simulink model "Integ_Model_Hepta_Runner"  (R2022a)
settings: configuration reference "VLS_Standard_Configuration" (kept outside this file)
libraries: simulink x1
settings Model: DataDictionary=Hepta_Integrated_SLDD.sldd  Creator=ahashem  LastModifiedBy=yli69
settings ConfigSetRef: SourceName=VLS_Standard_Configuration

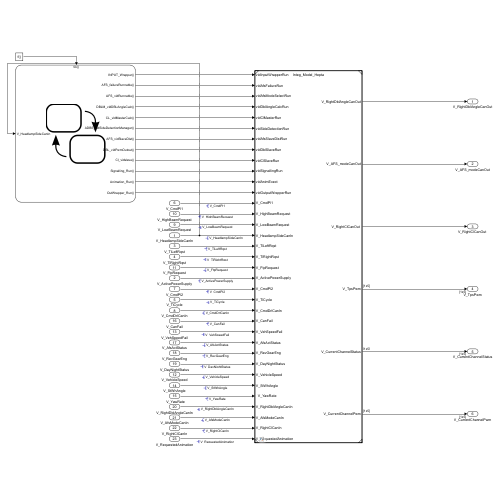
[thumbnail: Simulink's stored preview of the top-level diagram]
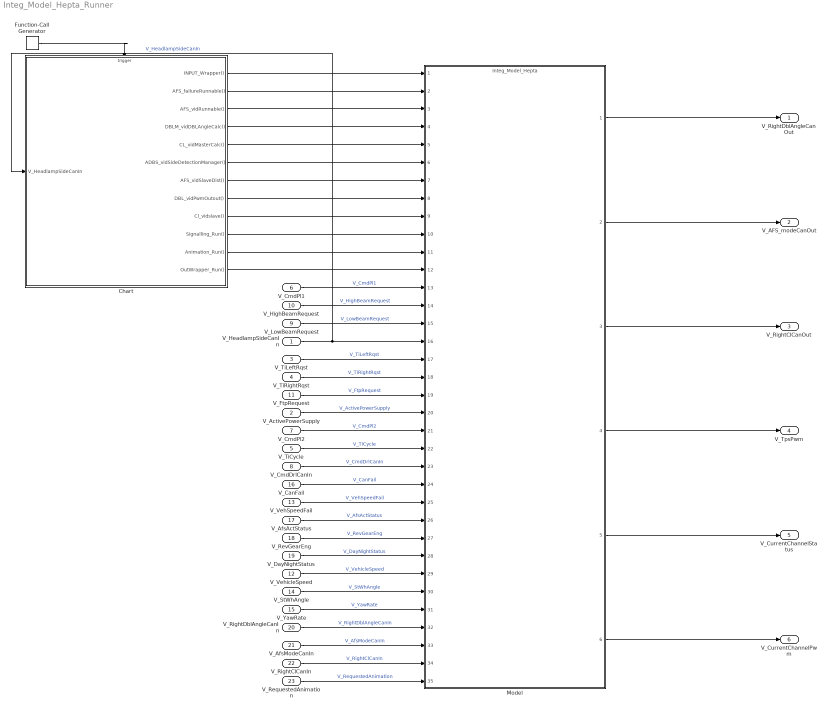
== system Integ_Model_Hepta_Runner ==
  V_HeadlampSideCanIn : Inport
  V_ActivePowerSupply : Inport  Port=2
  V_TiLeftRqst : Inport  Port=3
  V_TiRightRqst : Inport  Port=4
  V_TiCycle : Inport  Port=5
  V_CmdPl1 : Inport  Port=6
  V_CmdPl2 : Inport  Port=7
  V_CmdDrlCanIn : Inport  Port=8
  V_LowBeamRequest : Inport  Port=9
  V_HighBeamRequest : Inport  Port=10
  V_FtpRequest : Inport  Port=11
  V_VehicleSpeed : Inport  Port=12
  V_VehSpeedFail : Inport  Port=13
  V_StWhAngle : Inport  Port=14
  "  V_YawRate" : Inport  Port=15
  V_CanFail : Inport  Port=16
  V_AfsActStatus : Inport  Port=17
  V_RevGearEng : Inport  Port=18
  V_DayNightStatus : Inport  Port=19
  V_RightDblAngleCanIn : Inport  Port=20
  V_AfsModeCanIn : Inport  Port=21
  V_RightClCanIn : Inport  Port=22
  V_RequestedAnimation : Inport  Port=23
  Chart : Stateflow chart  TreatAsAtomicUnit=on
  Function-Call Generator : simulink/Ports & Subsystems/Function-Call Generator  sample_time=0.02  numberOfIterations=1  DisallowWideOutput=off
  Model : ModelReference  ModelNameDialog=Integ_Model_Hepta.slx  SimulationMode=Normal  ScheduleRates=on  ModelReferenceVersion=4.16
  V_RightDblAngleCanOut : Outport  VectorParamsAs1DForOutWhenUnconnected=off
  V_AFS_modeCanOut : Outport  Port=2  VectorParamsAs1DForOutWhenUnconnected=off
  "V_RightClCanOut " : Outport  Port=3  VectorParamsAs1DForOutWhenUnconnected=off
  V_TpsPwm : Outport  Port=4
  V_CurrentChannelStatus : Outport  Port=5
  V_CurrentChannelPwm : Outport  Port=6
  wires:
  Function-Call Generator/1 -> Chart/Trigger
  Chart/1(INPUT_Wrapper()) -> Model/1
  Chart/2(AFS_failureRunnable()) -> Model/2
  Chart/3(AFS_vidRunnable()) -> Model/3
  Chart/4(DBLM_vidDBLAngleCalc()) -> Model/4
  Chart/5(CL_vidMasterCalc()) -> Model/5
  Chart/6(ADBS_vidSideDetectionManager()) -> Model/6
  Chart/7(AFS_vidSlaveDist()) -> Model/7
  Chart/8(DBL_vidPwmOutout()) -> Model/8
  Chart/9(Cl_vidslave()) -> Model/9
  Chart/10(Signalling_Run()) -> Model/10
  Chart/11(Animation_Run()) -> Model/11
  V_HeadlampSideCanIn/1 -> Model/16, Chart/1(V_HeadlampSideCanIn)  "V_HeadlampSideCanIn"
  Model/1 -> V_RightDblAngleCanOut/1
  Model/2 -> V_AFS_modeCanOut/1
  Model/3 -> "V_RightClCanOut "/1
  Model/4 -> V_TpsPwm/1
  Model/5 -> V_CurrentChannelStatus/1
  Model/6 -> V_CurrentChannelPwm/1
  Chart/12(OutWrapper_Run()) -> Model/12
  V_CmdPl1/1 -> Model/13  "V_CmdPl1"
  V_HighBeamRequest/1 -> Model/14  "V_HighBeamRequest"
  V_LowBeamRequest/1 -> Model/15  "V_LowBeamRequest"
  V_TiLeftRqst/1 -> Model/17  "V_TiLeftRqst"
  V_TiRightRqst/1 -> Model/18  "V_TiRightRqst"
  V_FtpRequest/1 -> Model/19  "V_FtpRequest"
  V_ActivePowerSupply/1 -> Model/20  "V_ActivePowerSupply"
  V_CmdPl2/1 -> Model/21  "V_CmdPl2"
  V_TiCycle/1 -> Model/22  "V_TiCycle"
  V_CmdDrlCanIn/1 -> Model/23  "V_CmdDrlCanIn"
  V_CanFail/1 -> Model/24  "V_CanFail"
  V_VehSpeedFail/1 -> Model/25  "V_VehSpeedFail"
  V_AfsActStatus/1 -> Model/26  "V_AfsActStatus"
  V_RevGearEng/1 -> Model/27  "V_RevGearEng"
  V_DayNightStatus/1 -> Model/28  "V_DayNightStatus"
  V_VehicleSpeed/1 -> Model/29  "V_VehicleSpeed"
  V_StWhAngle/1 -> Model/30  "V_StWhAngle"
  "  V_YawRate"/1 -> Model/31  "V_YawRate"
  V_RightDblAngleCanIn/1 -> Model/32  "V_RightDblAngleCanIn"
  V_AfsModeCanIn/1 -> Model/33  "V_AfsModeCanIn"
  V_RightClCanIn/1 -> Model/34  "V_RightClCanIn"
  V_RequestedAnimation/1 -> Model/35  "V_RequestedAnimation"

== stateflow chart Integ_Model_Hepta_Runner/Chart ==
  state Scheduler_Master
    on every(2,tik):
    send(INPUT_Wrapper);
    on every(2,tik):
    send(AFS_failureRunnable);
    on every(2,tik):
    send(AFS_vidRunnable);
    on every(2,tik):
    send(DBLM_vidDBLAngleCalc);
    on every(2,tik):
    send(CL_vidMasterCalc);
    on every(2,tik):
    send(ADBS_vidSideDetectionManager);
    on every(2,tik):
    send(AFS_vidSlaveDist);
    on every(2,tik):
    send(DBL_vidPwmOutout);
    on every(2,tik):
    send(Cl_vidslave);
    on every(2,tik):
    send(Signalling_Run);
    on every(5,tik):
    send(Animation_Run);
    on every(2,tik):
    send(OutWrapper_Run);
  state Scheduler_Slave
    on every(2,tik):
    send(INPUT_Wrapper);
    on every(2,tik):
    send(ADBS_vidSideDetectionManager);
    on every(2,tik):
    send(AFS_vidSlaveDist);
    on every(2,tik):
    send(DBL_vidPwmOutout);
    on every(2,tik):
    send(Cl_vidslave);
    on every(2,tik):
    send(Signalling_Run);
    on every(5,tik):
    send(Animation_Run);
    on every(2,tik):
    send(OutWrapper_Run);
  (default) -> (junction 44)
  (junction 44) -> Scheduler_Slave [order 1] : [V_HeadlampSideCanIn]
  (junction 44) -> Scheduler_Master [order 2]
  Scheduler_Master -> Scheduler_Slave : [V_HeadlampSideCanIn]
  Scheduler_Slave -> Scheduler_Master : [V_HeadlampSideCanIn==0]
  data: V_HeadlampSideCanIn input
  events: INPUT_Wrapper output FUNCTION_CALL_EVENT; AFS_failureRunnable output FUNCTION_CALL_EVENT; AFS_vidRunnable output FUNCTION_CALL_EVENT; DBLM_vidDBLAngleCalc output FUNCTION_CALL_EVENT; CL_vidMasterCalc output FUNCTION_CALL_EVENT; ADBS_vidSideDetectionManager output FUNCTION_CALL_EVENT; AFS_vidSlaveDist output FUNCTION_CALL_EVENT; DBL_vidPwmOutout output FUNCTION_CALL_EVENT; Cl_vidslave output FUNCTION_CALL_EVENT; Signalling_Run output FUNCTION_CALL_EVENT; Animation_Run output FUNCTION_CALL_EVENT; tik input FUNCTION_CALL_EVENT; OutWrapper_Run output FUNCTION_CALL_EVENT
